simulink model "CONVERTER_SIMULATION"  (R2024a)
settings: Solver=VariableStepAuto  StartTime=0.0  StopTime=.03  RelTol=1e-3
undefined symbols (not defined in the file): Ion, Lithium
libraries: spsCurrentMeasurementLib x5, spsVoltageMeasurementLib x5, spsDiodeLib x4, spsMosfetLib x4, spsSeriesRLCBranchLib x4, spsBatteryLib x2, spsLinearTransformerLib x1, sps_lib x1
settings Model: Creator=mubar  LastModifiedBy=mubar

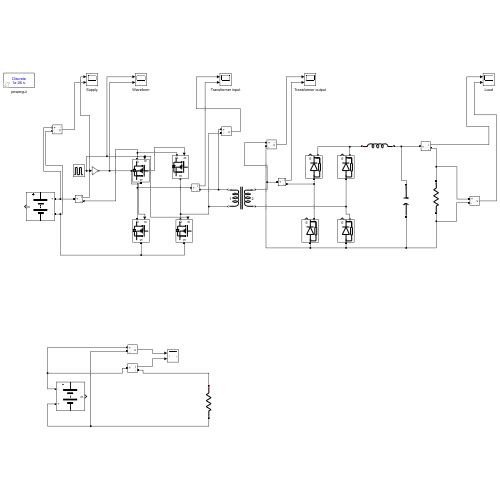
[thumbnail: Simulink's stored preview of the top-level diagram]
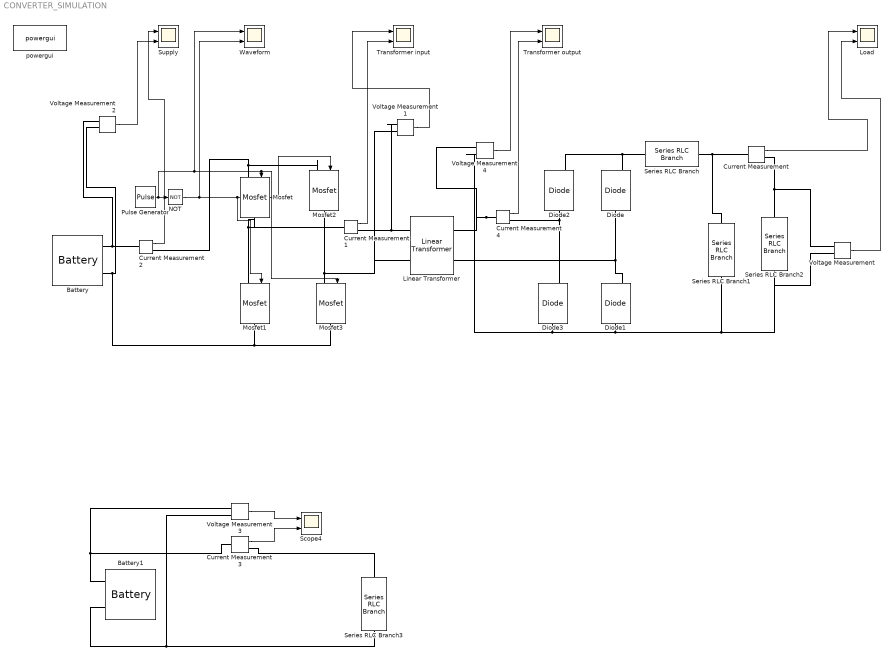
== system CONVERTER_SIMULATION ==
  Battery : spsBatteryLib/Battery  BatType=Lithium-Ion  ShowTempParam=off  ThermalPreset=no  ShowAgeParam=off  NomV=20  NomQ=100  SOC=100  Batt_Tr=1  PresetModel=on  MaxQ=100  MinV=15  FullV=23.2797  Dis_rate=43.4783  R=0.002  Normal_OP=90.4348  expZone="[21.6077      4.91304]"  current=[65 130 325]  Units=Time  Tci=20  NomT=20  T2=-30  MaxQ2=4.8  FullV2=7.1  Normal_OP2=5.655  expZone2="[6.58           1]"  Rca=0.6  ti=2000  Dp=0  Neq0=0  Tsim=1e6  Ta1=25  Qeol=5.4*0.9  Reol=0.013333*1.2  Char_age=[2.3478, 3]  Dis_age=[2.3478, 10]  N1=1500  N2=10500  N3=1000  N4=1400  Ta2=45  N5=950
  Battery1 : spsBatteryLib/Battery  BatType=Lithium-Ion  ShowTempParam=off  ThermalPreset=no  ShowAgeParam=off  NomV=12  NomQ=100  SOC=100  Batt_Tr=1  PresetModel=on  MaxQ=100  MinV=9  FullV=13.9678  Dis_rate=43.4783  R=0.0012  Normal_OP=90.4348  expZone="[12.9646      4.91304]"  current=[65 130 325]  Units=Time  Tci=20  NomT=20  T2=-30  MaxQ2=4.8  FullV2=7.1  Normal_OP2=5.655  expZone2="[6.58           1]"  Rca=0.6  ti=2000  Dp=0  Neq0=0  Tsim=1e6  Ta1=25  Qeol=5.4*0.9  Reol=0.013333*1.2  Char_age=[2.3478, 3]  Dis_age=[2.3478, 10]  N1=1500  N2=10500  N3=1000  N4=1400  Ta2=45  N5=950
  Current Measurement{,1..4} (5 alike) : spsCurrentMeasurementLib/Current Measurement  PhasorSimulation=off  OutputType=Complex  PSBequivalent=0
  Diode{,1..3} (4 alike) : spsDiodeLib/Diode  Ron=0.001  Lon=0  Vf=1  IC=0  UseSnubber=0  Rs=500  Cs=250e-9  Measurements=on
  Linear Transformer : spsLinearTransformerLib/Linear Transformer  UNITS=SI  NominalPower=[ 1000 300]  winding1="[20  0.159 20e-6]"  winding2=[400 0.819 50.3e-3]  ThreeWindings=off  winding3=[3.15e+05 0.7938 0.084225]  RmLm=[0.04 6.4e-3]  Measurements=None  DataType=on
  Load : Scope  NumInputPorts=2
  Mosfet{,1..3} (4 alike) : spsMosfetLib/Mosfet  Ron=0.1  Lon=0  Rd=0.01  Vfd=0  IC=0  Rs=1e5  Cs=inf  Measurements=off
  NOT : Logic  Operator=NOT  IconShape=distinctive  AllPortsSameDT=off  OutDataTypeStr=boolean
  Pulse Generator : DiscretePulseGenerator  PulseType=Time based  Period=1/30000  PulseWidth=50  VectorParams1D=off
  Scope4 : Scope  NumInputPorts=2
  Series RLC Branch : spsSeriesRLCBranchLib/Series RLC Branch  LConnTagsString=__new0  RConnTagsString=__new0  BranchType=L  Resistance=1  Inductance=1.2e-3  SetiL0=off  InitialCurrent=0  Capacitance=1e-6  Setx0=off  InitialVoltage=0  Measurements=None
  Series RLC Branch1 : spsSeriesRLCBranchLib/Series RLC Branch  LConnTagsString=__new0  RConnTagsString=__new0  BranchType=C  Resistance=1  Inductance=1e-3  SetiL0=off  InitialCurrent=0  Capacitance=470e-6  Setx0=on  InitialVoltage=5  Measurements=None
  Series RLC Branch2 : spsSeriesRLCBranchLib/Series RLC Branch  LConnTagsString=__new0  RConnTagsString=__new0  BranchType=R  Resistance=0.1  Inductance=50e-3  SetiL0=off  InitialCurrent=0  Capacitance=1e-6  Setx0=off  InitialVoltage=0  Measurements=None
  Series RLC Branch3 : spsSeriesRLCBranchLib/Series RLC Branch  LConnTagsString=__new0  RConnTagsString=__new0  BranchType=R  Resistance=2  Inductance=1e-3  SetiL0=off  InitialCurrent=0  Capacitance=1e-6  Setx0=off  InitialVoltage=0  Measurements=None
  Supply : Scope  NumInputPorts=2
  Transformer input : Scope  NumInputPorts=2
  Transformer output : Scope  NumInputPorts=2
  Voltage Measurement{,1..4} (5 alike) : spsVoltageMeasurementLib/Voltage Measurement  PhasorSimulation=off  OutputType=Complex  PSBequivalent=0
  Waveform : Scope  NumInputPorts=2
  powergui : sps_lib/powergui  Priority=1  SimulationMode=Discrete  SampleTime=1e-6  frequency=60  Iterations=50  frequencyindice=0  Pbase=100e6  ErrMax=1e-4  UnitsV=kV  UnitsW=MW  buscounter=0  FunctionMessages=off  echomessages=off  EnableUseOfTLC=off  CurrentSourceSwitches=off  DisableSnubberDevices=off  DisableRonSwitches=off  DisableVfSwitches=off  DisplayEquations=off  AutomaticDiscreteSolvers=off  SolverType=Tustin/Backward Euler (TBE)  Interpol=off  ExternalGateDelay=off  methode=off  Ts=100  x0status=blocks  SPID=on  SwTol=0  HookPort=off  NonlinearTolerance=1e-4  nMaxIteration=100  ContinueOnMaxIteration=off  RestoreLinks=warning  ResistiveCurrentMeasurement=off  Frange=[0:2:500]  Ylog=off  Xlog=on  ShowGrid=off  save=off  variable=ZData  structure=0  ZoomFFT=off  StartTime=0.0  cycles=1  DisplayStyle=1  fundamental=60  FreqAxis=off  MaxFrequency=1000  frequencyindicesteady=1  RmsSteady=1  display=off
  wires:
  Current Measurement/1 -> Load/1
  Voltage Measurement/1 -> Load/2
  Pulse Generator/1 -> Waveform/1, Mosfet/1, Mosfet3/1, NOT/1
  Voltage Measurement2/1 -> Supply/2
  Current Measurement2/1 -> Supply/1
  Voltage Measurement3/1 -> Scope4/1
  Current Measurement3/1 -> Scope4/2
  NOT/1 -> Waveform/2, Mosfet2/1, Mosfet1/1
  Current Measurement1/1 -> Transformer input/2
  Voltage Measurement1/1 -> Transformer input/1
  Voltage Measurement4/1 -> Transformer output/1
  Current Measurement4/1 -> Transformer output/2
  connections:
  Series RLC Branch/RConn1 -- Current Measurement/LConn1 -- Series RLC Branch1/LConn1
  Diode/LConn1 -- Diode1/RConn1 -- Linear Transformer/RConn2
  Diode3/RConn1 -- Current Measurement4/RConn1 -- Diode2/LConn1
  Diode3/LConn1 -- Series RLC Branch1/RConn1 -- Voltage Measurement/LConn2 -- Series RLC Branch2/RConn1 -- Diode1/LConn1 -- Voltage Measurement4/LConn2
  Diode2/RConn1 -- Series RLC Branch/LConn1 -- Diode/RConn1
  Series RLC Branch2/LConn1 -- Current Measurement/RConn1 -- Voltage Measurement/LConn1
  Battery1/LConn2 -- Voltage Measurement3/LConn1 -- Current Measurement3/LConn1
  Battery1/LConn1 -- Voltage Measurement3/LConn2 -- Series RLC Branch3/RConn1
  Current Measurement3/RConn1 -- Series RLC Branch3/LConn1
  Voltage Measurement1/LConn1 -- Linear Transformer/LConn1 -- Current Measurement1/RConn1
  Mosfet2/RConn1 -- Linear Transformer/LConn2 -- Voltage Measurement1/LConn2 -- Mosfet3/LConn1
  Battery/LConn2 -- Mosfet3/RConn1 -- Mosfet1/RConn1 -- Voltage Measurement2/LConn2
  Battery/LConn1 -- Voltage Measurement2/LConn1 -- Current Measurement2/LConn1
  Mosfet2/LConn1 -- Current Measurement2/RConn1 -- Mosfet/LConn1
  Mosfet/RConn1 -- Mosfet1/LConn1 -- Current Measurement1/LConn1
  Current Measurement4/LConn1 -- Linear Transformer/RConn1 -- Voltage Measurement4/LConn1
